simulink model "windTurbine"  (R2015b)
settings: Solver=FixedStepAuto  StartTime=0.0  StopTime=500  FixedStep=0.02  RelTol=1e-3
values from neighbouring files (symbols this model uses):
  beta = cpTable(1,2:37)    [nrel5MW.m]
  cpData = cpData*CpOpt/max(cpData(:))    [nrel5MW.m]
  CpOpt = max(cpData(:))    [nrel5MW.m]
  ctData = ctTable(2:21,2:37)    [nrel5MW.m]
  g = 9.80665    [runModel.m]
  Ki_pitch = rotor.I(3)*rotor.ratedSpeed*omega_phi^2/(-dP_dtheta(1))    [filterController.m]
  Ki_speed = omega_speed^2*rotor.I(3)    [filterController.m]
  Kp_pitch = 2*rotor.I(3)*rotor.ratedSpeed*zeta_phi*omega_phi/(-dP_dtheta(1))    [filterController.m]
  Kp_speed = 2*omega_speed*rotor.I(3)-hubBearingDamp    [filterController.m]
  omgM = 0.5*rotor.ratedSpeed    [filterController.m]
  rho_a = 1.225    [runModel.m]
  s = tf('s')    [runModel.m]
  sigmaV = 0.14*wind.speed    [runModel.m]
  theta_k = 8.7    [filterController.m]
  tipRatio = tipRatio+(tipRatioOpt-tipRatio(idx))    [nrel5MW.m]
  tipRatioOpt = 7.55    [nrel5MW.m]
undefined symbols (not defined in the file or in its folder): nacelle, rotor, tower, wind, wt, X, Y, Z
libraries: sm_lib x19, nesl_utility x16, cstblocks x2
settings Model: Creator=zhu  LastModifiedBy=zhu
settings ExplorerConfigSet: InternalSimMechanicsExplorerSettings="<ExplorerConfiguration><canonicalview>default</canonicalview><AnimationSetting><BasePlaybackSpeed>3</BasePlaybackSpeed><PlaybackSpeedFactor>1.0</PlaybackSpeedFactor></AnimationSetting><TilePanel><TileInfo><Tiles Columns=\"1\" Count=\"1\" Rows=\"1\"><Column Left=\"2\" Weight=\"1\"/><Column Left=\"1328\"/><Row Top=\"2\" Weight=\"1\"/><Row Top=\"769\"/><Tile Height=\"1\" Width=\"1\" X=\"0\" Y=\"0\"/></Tiles></TileInfo><SceneInfo><SceneViewer><BGColor><R>0.60000002384185791</R><G>0.60000002384185791</G><B>0.60000002384185791</B></BGColor><Camera><Position><X>-210.21893269604345</X><Y>-275.79049262918397</Y><Z>242.7874594457995</Z></Position><Center><X>-9.4287659580289347</X><Y>-12.411764241052573</Y><Z>46.341474445866716</Z></Center><Up><X>0.29745312815510411</X><Y>0.4146679029026798</Y><Z>0.85998381778556565</Z></Up><Left>-87.021720986708843</Left><Right>87.021720986708843</Right><Bottom>-87.364974639885148</Bottom><Top>87.364974639885148</Top></Camera></SceneViewer></SceneInfo></TilePanel></ExplorerConfiguration>"

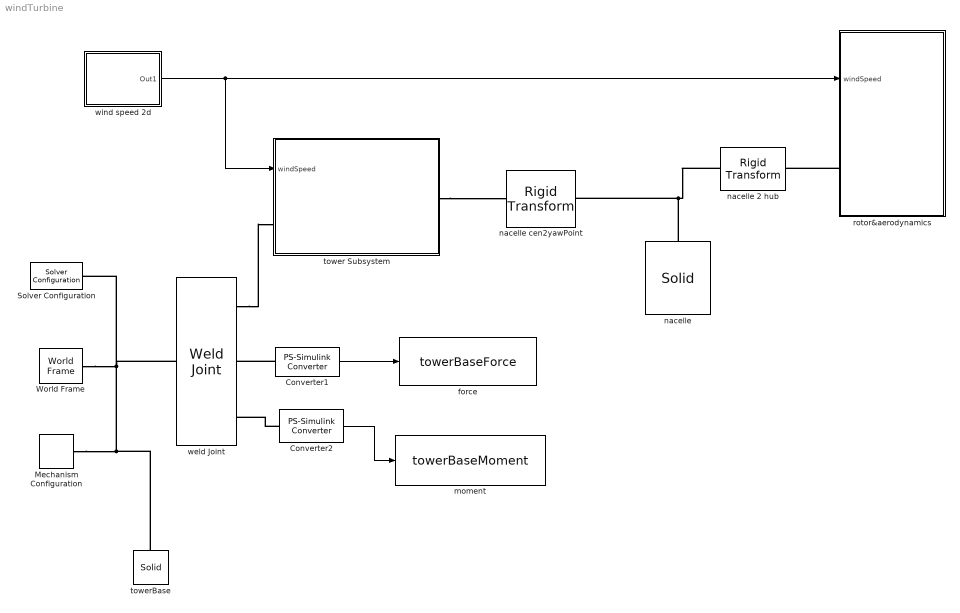
== system windTurbine ==
  Converter1 : nesl_utility/PS-Simulink Converter  PhysicalDomain=network_engine_domain  SubClassName=ps_output  LeftPortType=input  RightPortType=output  PseudoPeriodic=off  Frequencies=[]  Unit=1  AffineConversion=off
  Converter2 : nesl_utility/PS-Simulink Converter  PhysicalDomain=network_engine_domain  SubClassName=ps_output  LeftPortType=input  RightPortType=output  PseudoPeriodic=off  Frequencies=[]  Unit=1  AffineConversion=off
  Mechanism Configuration : sm_lib/Utilities/Mechanism Configuration  UniformGravity=Constant  GravityVector=[0 0 -g]  GravityUnits=m/s^2  LinearizationDelta=0.001  BlockFunction=simmechanics.library.utilities.mechanism_configuration
  Solver Configuration : nesl_utility/Solver Configuration  PhysicalDomain=network_engine_domain  SubClassName=solver  LeftPortType=input  RightPortType=generic  Accelerate=off  Tones=[]  Harmonics=[]  SimulateNoise=off  Profile=off  UseLocalSampling=off  EnableSwitchedLinearOptims=on  FrequencyDomain=off  UseCCode=off  RelTol=0.001  AbsTol=1e-06  MinStep=1e-09  ToWorkspace=off  RevertToSquareIcSolve=off  NumHomotopyIterations=100  PhasorMode=off  PhasorModeNumHarmonics=1  DoDC=off  ResidualTolerance=1e-09  UseLocalSolver=off  LocalSolverChoice=NE_BACKWARD_EULER_ADVANCER  LocalSolverSampleTime=0.001  DoFixedCost=off  MaxNonlinIter=3  MaxModeIter=2  LinearAlgebra=Sparse  DelaysMemoryBudget=1024  AutomaticFiltering=on  FilteringTimeConstant=0.001
  World Frame : sm_lib/Frames and Transforms/World Frame  BlockFunction=simmechanics.library.frames_transforms.world_frame
  force : ToWorkspace  VariableName=towerBaseForce  SaveFormat=Timeseries  SampleTime=-1
  moment : ToWorkspace  VariableName=towerBaseMoment  SaveFormat=Timeseries  SampleTime=-1
  nacelle : sm_lib/Body Elements/Solid  InertiaType=Custom  Mass=nacelle.m  MassUnits=kg  CenterOfMass=nacelle.com  CenterOfMassUnits=m  MomentsOfInertia=nacelle.I  MomentsOfInertiaUnits=kg*m^2  ProductsOfInertia=[0 0 0]  ProductsOfInertiaUnits=kg*m^2  DensityBased=on  Density=1000  DensityUnits=kg/(m^3)  DoExposeReferenceFrame=on  SerializedFrames=<Frames/>  GraphicType=FromGeometry  MarkerShape=Sphere  MarkerSize=10  GraphicVisPropType=SimpleVisualProperties  GraphicDiffuseColor=[0.2 1.0 1.0]  GraphicSpecularColor=[0.5 0.5 0.5 1.0]  GraphicAmbientColor=[0.15 0.15 0.15 1.0]  GraphicEmissiveColor=[0.0 0.0 0.0 1.0]  GraphicShininess=75  GraphicOpacity=1.0  GeometryShape=Brick  RectangleSize=[1 1]  RectangleSizeUnits=m  BrickDimensions=nacelle.dim  BrickDimensionUnits=m  CylinderRadius=1  CylinderRadiusUnits=m  CylinderLength=1  CylinderLengthUnits=m  SphereRadius=1  SphereRadiusUnits=m  EllipsoidRadii=[1 1 1]  EllipsoidRadiiUnits=m  ExtrusionCrossSection=[1 1; -1 1; -1 -1; 1 -1]  ExtrusionCrossSectionUnits=m  ExtrusionLength=1  ExtrusionLengthUnits=m  PolygonNumSides=3  PolygonOuterRadius=1  PolygonOuterRadiusUnits=m  ExtGeomFileType=STL  ExtGeomFileUnits=m  RevolutionCrossSection=[1 1; 1 -1; 2 -1; 2 1]  RevolutionCrossSectionUnits=m  RevolutionExtent=Full  RevolutionAngle=180  RevolutionAngleUnits=deg  BlockFunction=simmechanics.library.body_elements.solid
  nacelle 2 hub : sm_lib/Frames and Transforms/Rigid Transform  TranslationMethod=StandardAxis  TranslationLengthUnit=m  TranslationStandardAxis=+Z  TranslationStandardOffset=nacelle.dim(3)/2+1  TranslationCartesianOffset=[0 0 0]  TranslationROffset=0  TranslationROffsetUnits=m  TranslationZOffset=0  TranslationZOffsetUnits=m  TranslationThetaOffset=0  TranslationThetaOffsetUnits=deg  RotationMethod=None  RotationAngleUnits=deg  RotationStandardAxis=+Y  RotationAngle=90  RotationArbitraryAxis=[0 0 1]  FollAlignAxisA=+X  BaseAlignAxisA=+Y  FollAlignAxisB=+Y  BaseAlignAxisB=+Z  RotationSequenceAxes=FollowerAxes  RotationSequence=XYX  RotationSequenceAngles=[0 0 0]  RotationSequenceAnglesUnits=deg  RotationMatrix=[1 0 0; 0 1 0; 0 0 1]  BlockFunction=simmechanics.library.frames_transforms.rigid_transform
  nacelle cen2yawPoint : sm_lib/Frames and Transforms/Rigid Transform  TranslationMethod=StandardAxis  TranslationLengthUnit=m  TranslationStandardAxis=+Z  TranslationStandardOffset=0  TranslationCartesianOffset=[0 0 0]  TranslationROffset=0  TranslationROffsetUnits=m  TranslationZOffset=0  TranslationZOffsetUnits=m  TranslationThetaOffset=0  TranslationThetaOffsetUnits=deg  RotationMethod=StandardAxis  RotationAngleUnits=deg  RotationStandardAxis=+Y  RotationAngle=90  RotationArbitraryAxis=[0 0 1]  FollAlignAxisA=+X  BaseAlignAxisA=+Y  FollAlignAxisB=+Y  BaseAlignAxisB=+Z  RotationSequenceAxes=FollowerAxes  RotationSequence=XYX  RotationSequenceAngles=[0 0 0]  RotationSequenceAnglesUnits=deg  RotationMatrix=[1 0 0; 0 1 0; 0 0 1]  BlockFunction=simmechanics.library.frames_transforms.rigid_transform
  rotor&aerodynamics : Subsystem
  tower Subsystem : Subsystem
  towerBase : sm_lib/Body Elements/Solid  InertiaType=CalculateFromGeometry  Mass=1  MassUnits=kg  CenterOfMass=[0 0 0]  CenterOfMassUnits=m  MomentsOfInertia=[1 1 1]  MomentsOfInertiaUnits=kg*m^2  ProductsOfInertia=[0 0 0]  ProductsOfInertiaUnits=kg*m^2  DensityBased=off  Density=1000  DensityUnits=kg/(m^3)  DoExposeReferenceFrame=on  SerializedFrames=<Frames/>  GraphicType=FromGeometry  MarkerShape=Sphere  MarkerSize=10  GraphicVisPropType=SimpleVisualProperties  GraphicDiffuseColor=[0.5 0.5 0.5]  GraphicSpecularColor=[0.5 0.5 0.5 1.0]  GraphicAmbientColor=[0.15 0.15 0.15 1.0]  GraphicEmissiveColor=[0.0 0.0 0.0 1.0]  GraphicShininess=75  GraphicOpacity=1.0  GeometryShape=Cylinder  RectangleSize=[1 1]  RectangleSizeUnits=m  BrickDimensions=[1 1 1]  BrickDimensionUnits=m  CylinderRadius=100  CylinderRadiusUnits=m  CylinderLength=1  CylinderLengthUnits=m  SphereRadius=1  SphereRadiusUnits=m  EllipsoidRadii=[1 1 1]  EllipsoidRadiiUnits=m  ExtrusionCrossSection=[1 1; -1 1; -1 -1; 1 -1]  ExtrusionCrossSectionUnits=m  ExtrusionLength=1  ExtrusionLengthUnits=m  PolygonNumSides=3  PolygonOuterRadius=1  PolygonOuterRadiusUnits=m  ExtGeomFileType=STL  ExtGeomFileUnits=m  RevolutionCrossSection=[1 1; 1 -1; 2 -1; 2 1]  RevolutionCrossSectionUnits=m  RevolutionExtent=Full  RevolutionAngle=180  RevolutionAngleUnits=deg  BlockFunction=simmechanics.library.body_elements.solid
  weld Joint : sm_lib/Joints/Weld Joint  SenseConstraintForce=off  SenseConstraintForceX=off  SenseConstraintForceY=off  SenseConstraintForceZ=off  SenseConstraintTorque=off  SenseConstraintTorqueX=off  SenseConstraintTorqueY=off  SenseConstraintTorqueZ=off  SenseTotalForce=on  SenseTotalForceX=off  SenseTotalForceY=off  SenseTotalForceZ=off  SenseTotalTorque=on  SenseTotalTorqueX=off  SenseTotalTorqueY=off  SenseTotalTorqueZ=off  CompositeWrenchDir=FollowerOnBase  CompositeWrenchFrame=BaseFrame  BlockFunction=simmechanics.library.joints.weld_joint
  wind speed 2d : Subsystem
  wires:
  wind speed 2d/1(Out1) -> tower Subsystem/1("windSpeed "), rotor&aerodynamics/1("windSpeed ")
  Converter1/1 -> force/1
  Converter2/1 -> moment/1
  connections:
  nacelle 2 hub/LConn1 -- nacelle cen2yawPoint/LConn1 -- nacelle/RConn1
  Mechanism Configuration/RConn1 -- towerBase/RConn1 -- weld Joint/LConn1 -- Solver Configuration/RConn1 -- World Frame/RConn1
  rotor&aerodynamics/LConn1 -- nacelle 2 hub/RConn1
  tower Subsystem/RConn1 -- nacelle cen2yawPoint/RConn1
  weld Joint/RConn1 -- tower Subsystem/LConn1
  Converter1/LConn1 -- weld Joint/RConn2
  Converter2/LConn1 -- weld Joint/RConn3

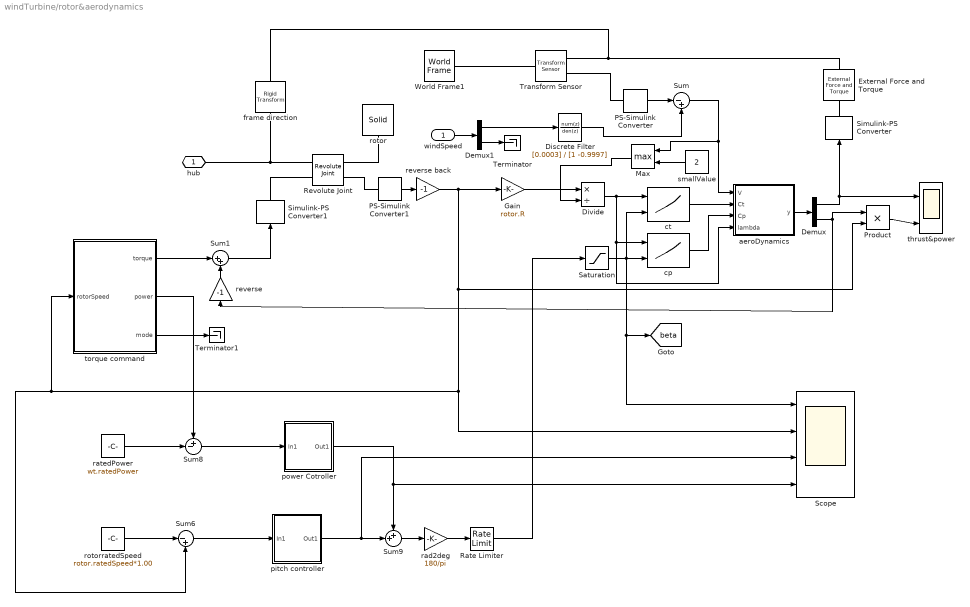
== system windTurbine/rotor&aerodynamics ==
  "windSpeed " : Inport
  Demux : Demux  Outputs=2
  Demux1 : Demux  Outputs=2
  Discrete Filter : DiscreteFilter  Numerator=[0.0003]  Denominator=[1 -0.9997]  SampleTime=0.02
  Divide : Product  Inputs=*/
  External Force and Torque : sm_lib/Forces and Torques/External Force and Torque  ForceResolutionFrame=AttachedFrame  EnableForceX=on  EnableForceY=off  EnableForceZ=off  EnableForce=off  TorqueResolutionFrame=AttachedFrame  EnableTorqueX=off  EnableTorqueY=off  EnableTorqueZ=off  EnableTorque=off  BlockFunction=simmechanics.library.forces_torques.external_force_torque
  Gain : Gain  Gain=rotor.R
  Max : MinMax  Function=max  Inputs=2
  PS-Simulink Converter : nesl_utility/PS-Simulink Converter  PhysicalDomain=network_engine_domain  SubClassName=ps_output  LeftPortType=input  RightPortType=output  PseudoPeriodic=off  Frequencies=[]  Unit=1  AffineConversion=off
  PS-Simulink Converter1 : nesl_utility/PS-Simulink Converter  PhysicalDomain=network_engine_domain  SubClassName=ps_output  LeftPortType=input  RightPortType=output  PseudoPeriodic=off  Frequencies=[]  Unit=1  AffineConversion=off
  Product : Product
  Rate Limiter : RateLimiter  RisingSlewLimit=8  FallingSlewLimit=-8  SampleTimeMode=inherited
  Revolute Joint : sm_lib/Joints/Revolute Joint  SenseConstraintForce=off  SenseConstraintForceX=off  SenseConstraintForceY=off  SenseConstraintForceZ=off  SenseConstraintTorque=off  SenseConstraintTorqueX=off  SenseConstraintTorqueY=off  SenseConstraintTorqueZ=off  SenseTotalForce=off  SenseTotalForceX=off  SenseTotalForceY=off  SenseTotalForceZ=off  SenseTotalTorque=off  SenseTotalTorqueX=off  SenseTotalTorqueY=off  SenseTotalTorqueZ=off  CompositeWrenchDir=FollowerOnBase  CompositeWrenchFrame=BaseFrame  EquilibriumPosition=0  EquilibriumPositionUnits=deg  SpringStiffness=0  SpringStiffnessUnits=N*m/deg  DampingCoefficient=0  DampingCoefficientUnits=N*m/(deg/s)  TorqueActuationMode=InputTorque  MotionActuationMode=ComputedMotion  SensePosition=off  SenseVelocity=on  SenseAcceleration=off  SenseTorqueForce=off  PositionTargetSpecify=off  PositionTargetPriority=High  PositionTargetValue=0  PositionTargetValueUnits=deg  VelocityTargetSpecify=on  VelocityTargetPriority=High  VelocityTargetValue=-rotor.ratedSpeed/6  VelocityTargetValueUnits=rad/s  BlockFunction=simmechanics.library.joints.revolute_joint
  Saturation : Saturate  UpperLimit=30  LowerLimit=0
  Scope : Scope  NumInputPorts=4
  Simulink-PS Converter : nesl_utility/Simulink-PS Converter  PhysicalDomain=network_engine_domain  SubClassName=ps_input  LeftPortType=input  RightPortType=output  PseudoPeriodic=off  Frequencies=[]  NoiseDistribution=none  NoiseParameters=[]  Unit=1  AffineConversion=off  InputFiltering=off  SimscapeFilterOrder=1  InputFilterTimeConstant=0.001  UdotUserProvided=1
  Simulink-PS Converter1 : nesl_utility/Simulink-PS Converter  PhysicalDomain=network_engine_domain  SubClassName=ps_input  LeftPortType=input  RightPortType=output  PseudoPeriodic=off  Frequencies=[]  NoiseDistribution=none  NoiseParameters=[]  Unit=1  AffineConversion=off  InputFiltering=off  SimscapeFilterOrder=1  InputFilterTimeConstant=0.001  UdotUserProvided=1
  Sum : Sum  Inputs=|-+
  Sum1 : Sum  Inputs=|++
  Sum6 : Sum  Inputs=|-+
  Sum8 : Sum  Inputs=+-|
  Sum9 : Sum  Inputs=++|
  Terminator : Terminator
  Terminator1 : Terminator
  Transform Sensor : sm_lib/Frames and Transforms/Transform Sensor  MeasurementFrame=World  SenseAngle=off  SenseAxis=off  SenseAngle1=off  SenseAngle2=off  SenseAngle3=off  SenseQ=off  SenseR=off  SenseOmegaX=off  SenseOmegaY=off  SenseOmegaZ=off  SenseOmega1=off  SenseOmega2=off  SenseOmega3=off  SenseQDot=off  SenseRDot=off  SenseAlphaX=off  SenseAlphaY=off  SenseAlphaZ=off  SenseAlpha1=off  SenseAlpha2=off  SenseAlpha3=off  SenseQDDot=off  SenseRDDot=off  SenseX=off  SenseY=off  SenseZ=off  SenseRad=off  SenseAzim=off  SenseDist=off  SenseInc=off  SenseXDot=on  SenseYDot=off  SenseZDot=off  SenseRadDot=off  SenseAzimDot=off  SenseDistDot=off  SenseIncDot=off  SenseXDDot=off  SenseYDDot=off  SenseZDDot=off  SenseRadDDot=off  SenseAzimDDot=off  SenseDistDDot=off  SenseIncDDot=off  BlockFunction=simmechanics.library.frames_transforms.transform_sensor
  World Frame1 : sm_lib/Frames and Transforms/World Frame  BlockFunction=simmechanics.library.frames_transforms.world_frame
  aeroDynamics : MATLAB Function  TreatAsAtomicUnit=on
  cp : Lookup_n-D  BreakpointsForDimension1=tipRatio  BreakpointsForDimension2=beta  Table=cpData  ExtrapMethod=Clip  UseLastTableValue=on  InternalRulePriority=Speed  RndMeth=Simplest  InputSameDT=on
  ct : Lookup_n-D  BreakpointsForDimension1=tipRatio  BreakpointsForDimension2=beta  Table=ctData  ExtrapMethod=Clip  UseLastTableValue=on  InternalRulePriority=Speed  RndMeth=Simplest  InputSameDT=on
  frame direction : sm_lib/Frames and Transforms/Rigid Transform  TranslationMethod=None  TranslationLengthUnit=m  TranslationStandardAxis=+Z  TranslationStandardOffset=0  TranslationCartesianOffset=[0 0 0]  TranslationROffset=0  TranslationROffsetUnits=m  TranslationZOffset=0  TranslationZOffsetUnits=m  TranslationThetaOffset=0  TranslationThetaOffsetUnits=deg  RotationMethod=StandardAxis  RotationAngleUnits=deg  RotationStandardAxis=+Y  RotationAngle=90  RotationArbitraryAxis=[0 0 1]  FollAlignAxisA=+X  BaseAlignAxisA=+Y  FollAlignAxisB=+Y  BaseAlignAxisB=+Z  RotationSequenceAxes=FollowerAxes  RotationSequence=XYX  RotationSequenceAngles=[0 0 0]  RotationSequenceAnglesUnits=deg  RotationMatrix=[1 0 0; 0 1 0; 0 0 1]  BlockFunction=simmechanics.library.frames_transforms.rigid_transform
  pitch controller : Subsystem
  power Cotroller : Subsystem
  rad2deg : Gain  Gain=180/pi
  ratedPower : Constant  Value=wt.ratedPower
  reverse : Gain  Gain=-1
  reverse back : Gain  Gain=-1
  rotor : sm_lib/Body Elements/Solid  InertiaType=Custom  Mass=rotor.m  MassUnits=kg  CenterOfMass=rotor.com  CenterOfMassUnits=m  MomentsOfInertia=rotor.I  MomentsOfInertiaUnits=kg*m^2  ProductsOfInertia=[0 0 0]  ProductsOfInertiaUnits=kg*m^2  DensityBased=on  Density=1000  DensityUnits=kg/(m^3)  DoExposeReferenceFrame=on  SerializedFrames=<Frames/>  GraphicType=FromGeometry  MarkerShape=Sphere  MarkerSize=10  GraphicVisPropType=SimpleVisualProperties  GraphicDiffuseColor=[0.6 0.8 1.0]  GraphicSpecularColor=[0.5 0.5 0.5 1.0]  GraphicAmbientColor=[0.15 0.15 0.15 1.0]  GraphicEmissiveColor=[0.0 0.0 0.0 1.0]  GraphicShininess=75  GraphicOpacity=1.0  GeometryShape=FromFile  RectangleSize=[1 1]  RectangleSizeUnits=m  BrickDimensions=[1 1 1]  BrickDimensionUnits=m  CylinderRadius=1  CylinderRadiusUnits=m  CylinderLength=1  CylinderLengthUnits=m  SphereRadius=1  SphereRadiusUnits=m  EllipsoidRadii=[1 1 1]  EllipsoidRadiiUnits=m  ExtrusionCrossSection=[1 1; -1 1; -1 -1; 1 -1]  ExtrusionCrossSectionUnits=m  ExtrusionLength=1  ExtrusionLengthUnits=m  PolygonNumSides=3  PolygonOuterRadius=1  PolygonOuterRadiusUnits=m  ExtGeomFileType=STL  ExtGeomFileName=blade.stl  ExtGeomFileUnits=m  RevolutionCrossSection=[1 1; 1 -1; 2 -1; 2 1]  RevolutionCrossSectionUnits=m  RevolutionExtent=Full  RevolutionAngle=180  RevolutionAngleUnits=deg  BlockFunction=simmechanics.library.body_elements.solid
  rotorratedSpeed : Constant  Value=rotor.ratedSpeed*1.00
  smallValue : Constant  Value=2
  thrust&power : Scope  NumInputPorts=2
  torque command : Subsystem
  hub : PMIOPort  Port=1  Side=Left
  tag scope: beta=global
  wires:
  Max/1 -> Divide/2
  ct/1 -> aeroDynamics/2(Ct)
  cp/1 -> aeroDynamics/3(Cp)
  Gain/1 -> Divide/1
  Divide/1 -> ct/1, cp/1, aeroDynamics/4(lambda)
  PS-Simulink Converter/1 -> Sum/1
  Sum/1 -> aeroDynamics/1(V), Max/1
  PS-Simulink Converter1/1 -> reverse back/1
  Demux/2 -> Product/1, reverse/1
  aeroDynamics/1(y) -> Demux/1
  Product/1 -> thrust&power/2
  Demux/1 -> Simulink-PS Converter/1, thrust&power/1
  smallValue/1 -> Max/2
  "windSpeed "/1 -> Demux1/1
  Demux1/1 -> Discrete Filter/1
  Demux1/2 -> Terminator/1
  reverse/1 -> Sum1/2
  Sum1/1 -> Simulink-PS Converter1/1
  Discrete Filter/1 -> Sum/2
  torque command/1(torque) -> Sum1/1
  Sum6/1 -> pitch controller/1(In1)
  rotorratedSpeed/1 -> Sum6/1
  reverse back/1 -> Gain/1, Scope/2, torque command/1(rotorSpeed), Sum6/2, Product/2
  ratedPower/1 -> Sum8/2
  torque command/2(power) -> Sum8/1
  pitch controller/1(Out1) -> Scope/3, Sum9/2
  power Cotroller/1(Out1) -> Sum9/1, Scope/4
  Saturation/1 -> [beta], Scope/1, cp/2, ct/2
  Sum8/1 -> power Cotroller/1(In1)
  Sum9/1 -> rad2deg/1
  rad2deg/1 -> Rate Limiter/1
  Rate Limiter/1 -> Saturation/1
  torque command/3(mode) -> Terminator1/1
  connections:
  Revolute Joint/RConn2 -- PS-Simulink Converter1/LConn1
  PS-Simulink Converter/LConn1 -- Transform Sensor/RConn2
  Revolute Joint/LConn2 -- Simulink-PS Converter1/RConn1
  rotor/RConn1 -- Revolute Joint/RConn1
  Simulink-PS Converter/RConn1 -- External Force and Torque/LConn1
  frame direction/RConn1 -- Transform Sensor/RConn1 -- External Force and Torque/RConn1
  hub/RConn1 -- frame direction/LConn1 -- Revolute Joint/LConn1
  Transform Sensor/LConn1 -- World Frame1/RConn1

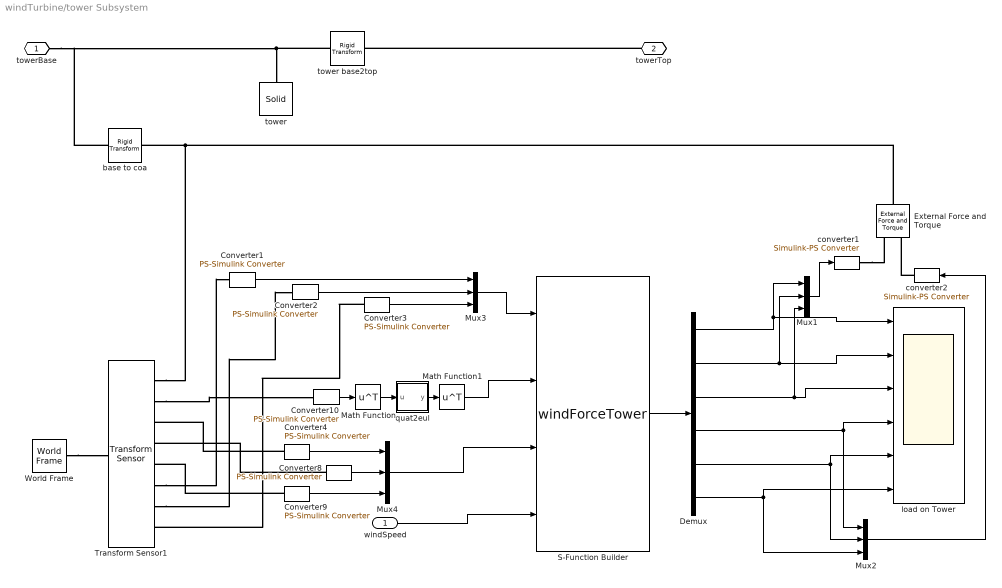
== system windTurbine/tower Subsystem ==
  "windSpeed " : Inport
  Converter{1..4,8..10} (7 alike) : nesl_utility/PS-Simulink Converter  PhysicalDomain=network_engine_domain  SubClassName=ps_output  LeftPortType=input  RightPortType=output  PseudoPeriodic=off  Frequencies=[]  Unit=1  AffineConversion=off
  Demux : Demux  Outputs=6
  External Force and Torque : sm_lib/Forces and Torques/External Force and Torque  ForceResolutionFrame=World  EnableForceX=off  EnableForceY=off  EnableForceZ=off  EnableForce=on  TorqueResolutionFrame=World  EnableTorqueX=off  EnableTorqueY=off  EnableTorqueZ=off  EnableTorque=on  BlockFunction=simmechanics.library.forces_torques.external_force_torque
  Math Function : Math  Operator=transpose  SaturateOnIntegerOverflow=on
  Math Function1 : Math  Operator=transpose  SaturateOnIntegerOverflow=on
  Mux{1..4} (4 alike) : Mux  Inputs=3
  S-Function Builder : S-Function  InitFcn=try, set_param(gcb,'FunctionName','windForceTower'), end  FunctionName=windForceTower  Parameters=tower.effR,tower.H,wind.alpha,rho_a,tower.cd,tower.CoA  SFunctionModules=windForceTower_wrapper  SFunctionDeploymentMode=off  EnableBusSupport=off  mask(S-Function Builder){}
      mask help: Simulink:masks:SFunctionBuilder_MD
      mask init:
      | val = [[.9  0.75 0.75 1 1 .9 .9 1]',[1 1 0.75 0.75 .9 .9 1 .9]'];try , sys = get_param(gcb,'SfunBuilderFcnName');if isempty(sys), sys = get_param(gcb,'FunctionName'); end,catch, sys = get_param(gcb,'FunctionName'); end
      settings: CopyFcn=set_param(gcbh,'LinkStatus','none')  PreSaveFcn=try, set_param(gcb,'FunctionName','windForceTower'), end  OpenFcn=sfunctionwizard(gcbh)
      mask Display: plot(val(:,1),val(:,2)),disp(sys), port_label('input',1,'dxcm'), port_label('input',2,'theta'), port_label('input',3,'omega'), port_label('input',4,'windSpeed'), port_label('output',1,'y0')
  Transform Sensor1 : sm_lib/Frames and Transforms/Transform Sensor  MeasurementFrame=World  SenseAngle=off  SenseAxis=off  SenseAngle1=off  SenseAngle2=off  SenseAngle3=off  SenseQ=on  SenseR=off  SenseOmegaX=on  SenseOmegaY=on  SenseOmegaZ=on  SenseOmega1=off  SenseOmega2=off  SenseOmega3=off  SenseQDot=off  SenseRDot=off  SenseAlphaX=off  SenseAlphaY=off  SenseAlphaZ=off  SenseAlpha1=off  SenseAlpha2=off  SenseAlpha3=off  SenseQDDot=off  SenseRDDot=off  SenseX=off  SenseY=off  SenseZ=off  SenseRad=off  SenseAzim=off  SenseDist=off  SenseInc=off  SenseXDot=on  SenseYDot=on  SenseZDot=on  SenseRadDot=off  SenseAzimDot=off  SenseDistDot=off  SenseIncDot=off  SenseXDDot=off  SenseYDDot=off  SenseZDDot=off  SenseRadDDot=off  SenseAzimDDot=off  SenseDistDDot=off  SenseIncDDot=off  BlockFunction=simmechanics.library.frames_transforms.transform_sensor
  World Frame : sm_lib/Frames and Transforms/World Frame  BlockFunction=simmechanics.library.frames_transforms.world_frame
  base to coa : sm_lib/Frames and Transforms/Rigid Transform  TranslationMethod=StandardAxis  TranslationLengthUnit=m  TranslationStandardAxis=+Z  TranslationStandardOffset=tower.H/2  TranslationCartesianOffset=0  TranslationROffset=0  TranslationROffsetUnits=m  TranslationZOffset=0  TranslationZOffsetUnits=m  TranslationThetaOffset=0  TranslationThetaOffsetUnits=deg  RotationMethod=None  RotationAngleUnits=deg  RotationStandardAxis=+Z  RotationAngle=0.0  RotationArbitraryAxis=[0 0 1]  FollAlignAxisA=+X  BaseAlignAxisA=+Y  FollAlignAxisB=+Y  BaseAlignAxisB=+Z  RotationSequenceAxes=FollowerAxes  RotationSequence=XYX  RotationSequenceAngles=[0 0 0]  RotationSequenceAnglesUnits=deg  RotationMatrix=[1 0 0; 0 1 0; 0 0 1]  BlockFunction=simmechanics.library.frames_transforms.rigid_transform
  converter1 : nesl_utility/Simulink-PS Converter  PhysicalDomain=network_engine_domain  SubClassName=ps_input  LeftPortType=input  RightPortType=output  PseudoPeriodic=off  Frequencies=[]  NoiseDistribution=none  NoiseParameters=[]  Unit=1  AffineConversion=off  InputFiltering=off  SimscapeFilterOrder=1  InputFilterTimeConstant=0.001  UdotUserProvided=1
  converter2 : nesl_utility/Simulink-PS Converter  PhysicalDomain=network_engine_domain  SubClassName=ps_input  LeftPortType=input  RightPortType=output  PseudoPeriodic=off  Frequencies=[]  NoiseDistribution=none  NoiseParameters=[]  Unit=1  AffineConversion=off  InputFiltering=off  SimscapeFilterOrder=1  InputFilterTimeConstant=0.001  UdotUserProvided=1
  load on Tower : Scope  NumInputPorts=6
  quat2eul : MATLAB Function  TreatAsAtomicUnit=on
  tower : sm_lib/Body Elements/Solid  InertiaType=Custom  Mass=tower.m  MassUnits=kg  CenterOfMass=tower.com  CenterOfMassUnits=m  MomentsOfInertia=tower.I  MomentsOfInertiaUnits=kg*m^2  ProductsOfInertia=[0 0 0]  ProductsOfInertiaUnits=kg*m^2  DensityBased=on  Density=0  DensityUnits=kg/(m^3)  DoExposeReferenceFrame=on  SerializedFrames=<Frames/>  GraphicType=FromGeometry  MarkerShape=Sphere  MarkerSize=10  MarkerSizeUnits=m  GraphicVisPropType=SimpleVisualProperties  GraphicDiffuseColor=[1.0 1.0 1.0]  GraphicSpecularColor=[0.5 0.5 0.5 1.0]  GraphicAmbientColor=[0.15 0.15 0.15 1.0]  GraphicEmissiveColor=[0.0 0.0 0.0 1.0]  GraphicShininess=75  GraphicOpacity=1.0  GeometryShape=GeneralSolidOfRevolution  RectangleSize=[1 1]  RectangleSizeUnits=m  BrickDimensions=[1 1 1]  BrickDimensionUnits=m  CylinderRadius=1  CylinderRadiusUnits=m  CylinderLength=1  CylinderLengthUnits=m  SphereRadius=1  SphereRadiusUnits=m  EllipsoidRadii=[1 1 1]  EllipsoidRadiiUnits=m  ExtrusionCrossSection=[1 1; -1 1; -1 -1; 1 -1]  ExtrusionCrossSectionUnits=m  ExtrusionLength=1  ExtrusionLengthUnits=m  PolygonNumSides=3  PolygonOuterRadius=1  PolygonOuterRadiusUnits=m  ExtGeomFileType=STL  ExtGeomFileUnits=m  RevolutionCrossSection=tower.section  RevolutionCrossSectionUnits=m  RevolutionExtent=Full  RevolutionAngle=180  RevolutionAngleUnits=deg  BlockFunction=simmechanics.library.body_elements.solid
  tower base2top : sm_lib/Frames and Transforms/Rigid Transform  TranslationMethod=StandardAxis  TranslationLengthUnit=m  TranslationStandardAxis=+Z  TranslationStandardOffset=tower.H  TranslationCartesianOffset=[0 0 0]  TranslationROffset=0  TranslationROffsetUnits=m  TranslationZOffset=0  TranslationZOffsetUnits=m  TranslationThetaOffset=0  TranslationThetaOffsetUnits=deg  RotationMethod=None  RotationAngleUnits=deg  RotationStandardAxis=+Z  RotationAngle=0.0  RotationArbitraryAxis=[0 0 1]  FollAlignAxisA=+X  BaseAlignAxisA=+Y  FollAlignAxisB=+Y  BaseAlignAxisB=+Z  RotationSequenceAxes=FollowerAxes  RotationSequence=XYX  RotationSequenceAngles=[0 0 0]  RotationSequenceAnglesUnits=deg  RotationMatrix=[1 0 0; 0 1 0; 0 0 1]  BlockFunction=simmechanics.library.frames_transforms.rigid_transform
  towerBase : PMIOPort  Port=1  Side=Left
  towerTop : PMIOPort  Port=2  Side=Right
  wires:
  "windSpeed "/1 -> S-Function Builder/4
  Mux2/1 -> converter2/1
  Mux1/1 -> converter1/1
  S-Function Builder/1 -> Demux/1
  Demux/5 -> load on Tower/5, Mux2/2
  Demux/4 -> load on Tower/4, Mux2/1
  Demux/3 -> load on Tower/3, Mux1/3
  Demux/2 -> load on Tower/2, Mux1/2
  Demux/1 -> load on Tower/1, Mux1/1
  Math Function1/1 -> S-Function Builder/2
  Mux3/1 -> S-Function Builder/1
  Converter3/1 -> Mux3/3
  Converter2/1 -> Mux3/2
  Converter1/1 -> Mux3/1
  Converter10/1 -> Math Function/1
  quat2eul/1(y) -> Math Function1/1
  Math Function/1 -> quat2eul/1(u)
  Mux4/1 -> S-Function Builder/3
  Converter4/1 -> Mux4/1
  Converter8/1 -> Mux4/2
  Converter9/1 -> Mux4/3
  Demux/6 -> load on Tower/6, Mux2/3
  connections:
  towerTop/RConn1 -- tower base2top/RConn1
  converter2/RConn1 -- External Force and Torque/LConn2
  converter1/RConn1 -- External Force and Torque/LConn1
  Converter3/LConn1 -- Transform Sensor1/RConn8
  Transform Sensor1/RConn7 -- Converter2/LConn1
  Transform Sensor1/RConn6 -- Converter1/LConn1
  Transform Sensor1/RConn2 -- Converter10/LConn1
  World Frame/RConn1 -- Transform Sensor1/LConn1
  tower base2top/LConn1 -- base to coa/LConn1 -- towerBase/RConn1 -- tower/RConn1
  Transform Sensor1/RConn1 -- External Force and Torque/RConn1 -- base to coa/RConn1
  Converter4/LConn1 -- Transform Sensor1/RConn3
  Converter8/LConn1 -- Transform Sensor1/RConn4
  Converter9/LConn1 -- Transform Sensor1/RConn5

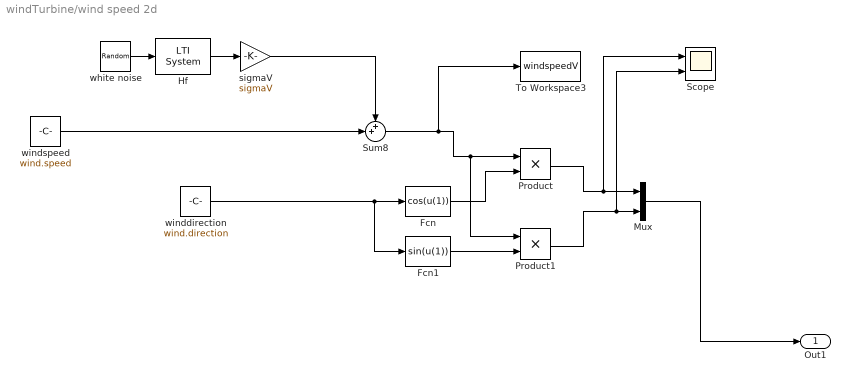
== system windTurbine/wind speed 2d ==
  Fcn : Fcn  Expr=cos(u(1))
  Fcn1 : Fcn  Expr=sin(u(1))
  Hf : cstblocks/LTI System  sys=Hf  IC=[]
  Mux : Mux  Inputs=2
  Product : Product
  Product1 : Product
  Scope : Scope  NumInputPorts=2
  Sum8 : Sum  Inputs=++|
  To Workspace3 : ToWorkspace  VariableName=windspeedV  SaveFormat=Timeseries  SampleTime=-1
  sigmaV : Gain  Gain=sigmaV
  white noise : RandomNumber  Seed=255  SampleTime=0.02
  winddirection : Constant  Value=wind.direction
  windspeed : Constant  Value=wind.speed
  Out1 : Outport
  wires:
  windspeed/1 -> Sum8/2
  Sum8/1 -> Product/1, Product1/1, To Workspace3/1
  white noise/1 -> Hf/1
  Hf/1 -> sigmaV/1
  Fcn/1 -> Product/2
  Product1/1 -> Scope/2, Mux/2
  Mux/1 -> Out1/1
  winddirection/1 -> Fcn/1, Fcn1/1
  Fcn1/1 -> Product1/2
  Product/1 -> Scope/1, Mux/1
  sigmaV/1 -> Sum8/1

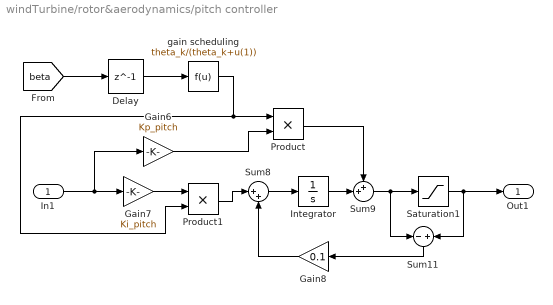
== system windTurbine/rotor&aerodynamics/pitch controller ==
  In1 : Inport
  Delay : Delay  DelayLength=1  InitialCondition=0
  Gain6 : Gain  Gain=Kp_pitch
  Gain7 : Gain  Gain=Ki_pitch
  Gain8 : Gain  Gain=0.1
  Integrator : Integrator
  Product : Product
  Product1 : Product
  Saturation1 : Saturate  UpperLimit=40  LowerLimit=0
  Sum11 : Sum  Inputs=-|+
  Sum8 : Sum  Inputs=|++
  Sum9 : Sum  Inputs=++|
  gain scheduling : Fcn  Expr=theta_k/(theta_k+u(1))
  Out1 : Outport
  wires:
  In1/1 -> Gain7/1, Gain6/1
  Saturation1/1 -> Sum11/2, Out1/1
  Sum8/1 -> Integrator/1
  Sum9/1 -> Sum11/1, Saturation1/1
  Integrator/1 -> Sum9/2
  Gain8/1 -> Sum8/2
  Sum11/1 -> Gain8/1
  Gain6/1 -> Product/2
  gain scheduling/1 -> Product/1, Product1/2
  Product/1 -> Sum9/1
  Gain7/1 -> Product1/1
  Product1/1 -> Sum8/1
  Delay/1 -> gain scheduling/1
  [beta] -> Delay/1

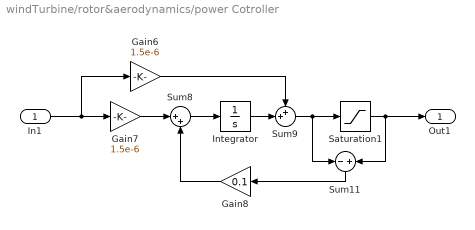
== system windTurbine/rotor&aerodynamics/power Cotroller ==
  In1 : Inport
  Gain6 : Gain  Gain=1.5e-6
  Gain7 : Gain  Gain=1.5e-6
  Gain8 : Gain  Gain=0.1
  Integrator : Integrator
  Saturation1 : Saturate  UpperLimit=15  LowerLimit=0
  Sum11 : Sum  Inputs=-|+
  Sum8 : Sum  Inputs=|++
  Sum9 : Sum  Inputs=++|
  Out1 : Outport
  wires:
  Sum11/1 -> Gain8/1
  Gain8/1 -> Sum8/2
  Integrator/1 -> Sum9/2
  Gain6/1 -> Sum9/1
  Sum9/1 -> Saturation1/1, Sum11/1
  Gain7/1 -> Sum8/1
  Sum8/1 -> Integrator/1
  Saturation1/1 -> Out1/1, Sum11/2
  In1/1 -> Gain6/1, Gain7/1

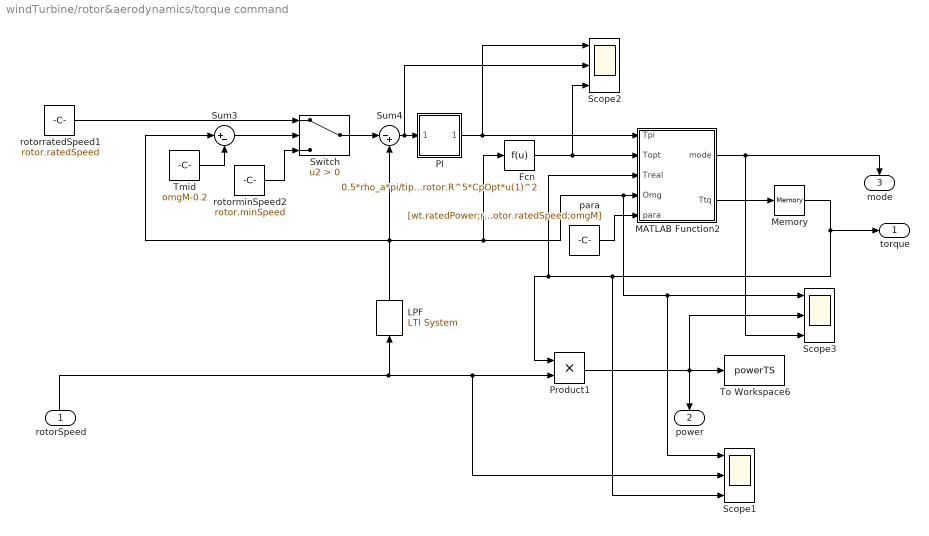
== system windTurbine/rotor&aerodynamics/torque command ==
  rotorSpeed : Inport
  Fcn : Fcn  Expr=0.5*rho_a*pi/tipRatioOpt^3*rotor.R^5*CpOpt*u(1)^2
  LPF : cstblocks/LTI System  sys=speedLPF4Ctrl  IC=[]
  MATLAB Function2 : MATLAB Function  TreatAsAtomicUnit=on
  Memory : Memory
  "PI " : Subsystem
  Product1 : Product
  Scope1 : Scope  NumInputPorts=3
  Scope2 : Scope  NumInputPorts=3
  Scope3 : Scope  NumInputPorts=3
  Sum3 : Sum  Inputs=|+-
  Sum4 : Sum  Inputs=|-+
  Switch : Switch  Criteria=u2 > Threshold
  Tmid : Constant  Value=omgM-0.2
  To Workspace6 : ToWorkspace  VariableName=powerTS  SaveFormat=Timeseries  SampleTime=-1
  para : Constant  Value=[wt.ratedPower;rotor.ratedSpeed;omgM]
  rotorminSpeed2 : Constant  Value=rotor.minSpeed
  rotorratedSpeed1 : Constant  Value=rotor.ratedSpeed
  torque : Outport
  power : Outport  Port=2
  mode : Outport  Port=3
  wires:
  Fcn/1 -> Scope2/3, MATLAB Function2/2(Topt)
  Sum4/1 -> Scope2/2, "PI "/1(In1)
  Product1/1 -> Scope3/2, power/1, To Workspace6/1
  Sum3/1 -> Switch/2
  para/1 -> MATLAB Function2/5(para)
  Memory/1 -> torque/1, Product1/1, MATLAB Function2/3(Treal), Scope1/3
  rotorminSpeed2/1 -> Switch/3
  rotorSpeed/1 -> Scope1/2, Product1/2, LPF/1
  Tmid/1 -> Sum3/2
  MATLAB Function2/2(Ttq) -> Memory/1
  MATLAB Function2/1(mode) -> mode/1, Scope3/3
  rotorratedSpeed1/1 -> Switch/1
  Switch/1 -> Sum4/1
  "PI "/1(Out1) -> Scope2/1, MATLAB Function2/1(Tpi)
  LPF/1 -> Sum4/2, Sum3/1, Scope1/1, Scope3/1, MATLAB Function2/4(Omg), Fcn/1

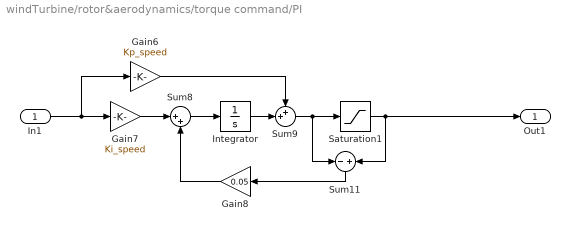
== system windTurbine/rotor&aerodynamics/torque command/PI  ==
  In1 : Inport
  Gain6 : Gain  Gain=Kp_speed
  Gain7 : Gain  Gain=Ki_speed
  Gain8 : Gain  Gain=0.05
  Integrator : Integrator
  Saturation1 : Saturate  UpperLimit=wt.ratedTorq  LowerLimit=0
  Sum11 : Sum  Inputs=-|+
  Sum8 : Sum  Inputs=|++
  Sum9 : Sum  Inputs=++|
  Out1 : Outport
  wires:
  In1/1 -> Gain7/1, Gain6/1
  Sum8/1 -> Integrator/1
  Gain7/1 -> Sum8/1
  Sum9/1 -> Sum11/1, Saturation1/1
  Gain6/1 -> Sum9/1
  Integrator/1 -> Sum9/2
  Gain8/1 -> Sum8/2
  Sum11/1 -> Gain8/1
  Saturation1/1 -> Out1/1, Sum11/2

== matlab function windTurbine/rotor&aerodynamics/torque command/MATLAB Function2 ==
  data: Tpi input; mode output; Topt input; Treal input; Omg input; para input; Ttq output
function [mode,Ttq] = fcn(Tpi,Topt,Treal,Omg,para)
% flag: 1->above rated flag
% mode: 5->Omg<Omg_mid, 6->Omg>Omg_mid, 2->Rated mode
Power_R = para(1);
Omg_R = para(2);
Omg_M = para(3);

Power = Treal * Omg;
speedMargin = 0.08;
mode=0;
Ttq=0;

if(Omg < Omg_M)
    mode = 5;
end
if(Omg >=Omg_M && Omg<=(1+speedMargin)*Omg_R)
    mode = 6;
end
if(Omg>(1+speedMargin)*Omg_R)
   mode = 2;
end

if(mode == 5)
    if(Tpi >= Topt)
        Ttq = Topt;
    else
        Ttq = Tpi;
    end
end
if(mode == 6)
    if(Tpi <= Topt)
        Ttq = Topt;
    else
        Ttq = Tpi;
    end
end

if(mode == 2)
    Ttq = Power_R/Omg_R; % constant torque
end

== matlab function windTurbine/tower Subsystem/quat2eul ==
  data: u input; y output
function y = fcn(u)
%#codegen

x = quat2eul(u);
y = [0 0 0];
y(1) = x(3);
y(2) = x(2);
y(3) = x(1);

== matlab function windTurbine/rotor&aerodynamics/aeroDynamics ==
  data: V input; y output; Ct input; Cp input; lambda input
function y  = fcn(V,Ct,Cp,lambda)
%#codegen
y=zeros(2,1);
rho_a = 1.225;
Rr = 63;
y(1)=0.5*rho_a*pi*Rr^2*Ct*V*abs(V);
if(lambda<0.2)
    Cq = Cp/0.2;
else
    Cq = Cp/lambda;
end
y(2)=0.5*rho_a*pi*Rr^3*Cq*V^2;
